simulink model "IEEE_9bus"  (R2023b)
settings: Solver=ode23tb  StartTime=0.0  StopTime=1  FixedStep=Ts  RelTol=1e-3
values from neighbouring files (symbols this model uses):
  N = 1    [IEEE_9bus_calc.m]
  Ts = 50e-6    (= 5e-05)    [IEEE_9bus_calc.m]
  Ws = 2*pi*f    (= 376.991118431)    [IEEE_9bus_calc.m]
undefined symbols (not defined in the file or in its folder): D1, Delta, DiscIntNeverNeededParam, SM, SYS
libraries: spsLoadFlowBusLib x9, spsabctodq0Lib x7, spsThreePhasePISectionLineLib x6, spsExcitationSystemLib x6, spsGenericPowerSystemStabilizerLib x6, spsHydraulicTurbineandGovernorLib x6, spsMultiBandPowerSystemStabilizerLib x6, spsThreePhaseVIMeasurementLib x5, spsThreePhaseSeriesRLCLoadLib x4, DQN_Lib x3, spsGroundLib x3, spsThreePhaseParallelRLCBranchLib x3
(part 1 of 3)
settings Model: Creator=z0034ktr  LastModifiedBy=rober
settings SolverCC: AlgebraicLoopSolver=TrustRegion  EnableFixedStepZeroCrossing=on
settings ModelReferenceCC: EnableRefExpFcnMdlSchedulingChecks=on

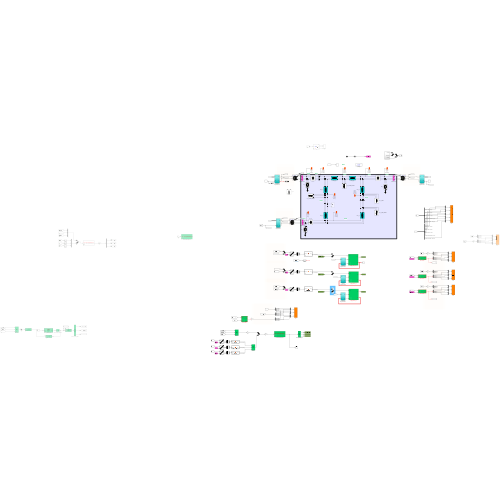
[thumbnail: Simulink's stored preview of the top-level diagram]
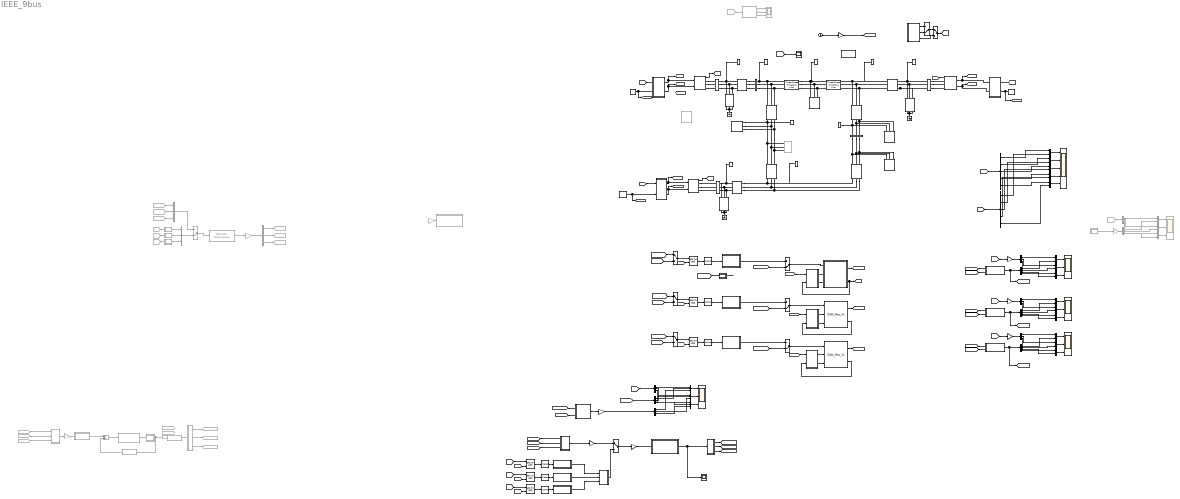
== system IEEE_9bus ==
  note: BUS7
  note: BUS7
  note: BUS2
  note: BUS8
  note: BUS9
  note: BUS3
  note: BUS6
  note: BUS4
  note: BUS5
  note: BUS1
  ABsel : Subsystem  Commented=on
  ABsel1 : Subsystem  Commented=on
  ABsel2 : Subsystem  Commented=on
  ABsel3 : Subsystem
  ABsel4 : Subsystem  Commented=on
  Add3 : Sum  Commented=on
  Bus Selector : BusSelector  OutputSignals="dq0 components.Stator voltage  vd (pu),dq0 components.Stator voltage  vq (pu),Mechanical.Rotor speed  wm  (pu),Mechanical.Rotor speed deviation  dw (pu),Output active power   Peo (pu)"
  Bus Selector1 : BusSelector  OutputSignals="Stator voltage  vd (pu),Stator voltage  vq (pu),Rotor speed  wm  (pu),Rotor speed deviation  dw (pu),Output active power   Peo (pu)"
  Clock : Clock
  Constant : Constant  Value=0.65694
  Constant1 : Constant  Value=0.825
  Constant2 : Constant  Value=0.425
  DQN_Mac1_V1 : Subsystem  mask{HRM=N, NomParam=[200E6  16500   60 ], reactVec=[ 1.305, 0.296, 0.252, 0.474, 0.243, 0.18 ], timeConstVec=[ 1.01, 0.053, 0.0513 ], Rs=2.8544e-3, Mech=[ 3.7 0  32], lfVec=[0.6569    0.3081    1.0000    1.5789   deg2rad(0)], Ts=Ts, SW=on, dbg=off, SMdbg=[]}
      mask prompts: HRM "Harmonic order:"; NomParam "Nominal power, line-to-line voltage, frequency [ Pn(VA)  Vn(Vrms)  fn(Hz) ]:"; reactVec "Reactances [ Xd  Xd'  Xd''  Xq  (Xq')  Xq''  Xl ] (pu):"; timeConstVec "[ Td'  Td''  (Tq')  Tq'' ] (s):"; Rs "Stator resistance Rs (pu):"; Mech "Inertia coefficient, friction factor, pole pairs [ H(s)  F(pu)  p()]:"; lfVec "Initial condition (P, Q, Vbus, Vf, angle) [1x6]:"; Ts "Integration timestep (s):"; SW "Method (dq - checked / abc - unchecked)"; dbg "Debug [external SM(RD) variable]"; SMdbg "Debug SM:"
      mask init:
      | SMRD = struct();
      | 
      |     SMRD.dwo = 0;
      | 
      |     SMRD.nState = numel(reactVec)-1;
      |     
      |     if(SMRD.nState>5)
      |         SMRD.RLinv   = zeros(6,6);
      |         SMRD.Linv    = zeros(6,6);
      |         SMRD.L       = zeros(6,6);
      |         SMRD.R       = zeros(6,6);
      |         W = zeros(6,6);
      |     else
      |         SMRD.RLinv   = zeros(5,5);
      |         SMRD.Linv    = zeros(5,5);
      |         SMRD.L       = zeros(5,5);
      |         SMRD.R       = zeros(5,5);
      |         W            = zeros(5,5);
      |     end
      | 
      |     SMRD.Rs      = Rs;
      | 
      |     SMRD.N       = 1;
      |     
      |     SMRD.H       = Mech(1);
      |     SMRD.F       = Mech(2);
      |     SMRD.p       = Mech(3);
      | 
      |     SMRD.Pn = NomParam(1);
      |     SMRD.Vn = NomParam(2);
      |     SMRD.fn = NomParam(3);
      |     
      |     
      |     Vb = SMRD.Vn*sqrt(2/3);
      |     Ib = sqrt(2/3)*SMRD.Pn/SMRD.Vn;
      |     
      |     
      |     Td_p    = timeConstVec(1);
      |     Td_pp   = timeConstVec(2);
      |     if(SMRD.nState>5)
      |         Tq_p    = timeConstVec(3);
      |         Tq_pp   = timeConstVec(4);
      |     else
      |         Tq_pp   = timeConstVec(3);
      |     end
      |     
      |     
      |     %Set the time constants in Lq(s)
      |     %See (eq. 7.2.14)
      |     
      |     wn=2*pi*SMRD.fn;
      |     SMRD.wn = wn;%Rated frequency in rad/sec
      |     %Implementation of the formulas in 
      |     
      |     % Xaq=1.165; %Mutual inductance
      |     % Ll=.188; %Stator leakage inductance
      |     
      |     %T5=0.0234;
      |     
      |     
      |     Xd      = reactVec(1);
      |     Xd_p    = reactVec(2);
      |     Xd_pp   = reactVec(3);
      |     Xq      = reactVec(4);
      | 
      | 
      |     if(SMRD.nState>5)
      |         Xq_p    = reactVec(5);
      |         Xq_pp   = reactVec(6);
      |         Xl      = reactVec(7);
      | 
      |         Tqo_p   = Tq_p * Xq/Xq_p;
      |         Tqo_pp  = Tq_pp * Xq_p/Xq_pp;
      |     else
      |         Xq_pp   = reactVec(5);
      |         Xl      = reactVec(6);
      |         Tqo_pp  = Tq_pp * Xq/Xq_pp;
      |     end
      | 
      | 
      |     Xad     = Xd-Xl; %Mutual inductance
      |     Xaq     = Xq-Xl; %Mutual inductance
      |     
      |     
      |     SMRD.Xd = Xd;
      |     SMRD.Xq = Xq;
      |     SMRD.Xl = Xl;
      |     SMRD.Xad = Xad;
      |     SMRD.Xaq = Xaq;
      |     
      |         
      |    
      |     LAM1 = sqrt(Xd^2*Xd_pp^2*(Td_p-Td_pp)^2+2*Td_p*Td_pp*Xd*Xd_p*Xd_pp*(Xd-2*Xd_p+Xd_pp)-2*Td_pp*Xd*Xd_p*Xd_pp*(Xd-Xd_p+Xd_pp)+Td_pp^2*Xd_pp^2*(Xd^2+Xd_pp^2));
      |     Tdo_p  = (Td_p*Xd*Xd_pp+LAM1+Td_pp*(Xd*Xd_p+Xd_p*Xd_pp-Xd*Xd_pp))/(2*Xd_p*Xd_pp);
      |     Tdo_pp = Xd*Td_p*Td_pp/(Xd_pp*Tdo_p);
      |     % 
      |     % Tqo_p   = Tq_p * Xq/Xq_p;
      |     % Tqo_pp  = Tq_pp * Xq_p/Xq_pp;
      | 
      | 
      |     % D-Axis
      |     a=SMRD.Xad*(Xd_p-SMRD.Xl)/(Xd-Xd_p);
      |     b=a*SMRD.Xad*(Xd_pp-SMRD.Xl)/(a*Xd+SMRD.Xl*SMRD.Xad-(a+SMRD.Xad)*Xd_pp);
      |     c=(b+a*SMRD.Xl*SMRD.Xad/(SMRD.Xl*SMRD.Xad+a*Xd))/Td_pp;
      |     
      |     T5 = b/c;
      | 
      |     if(1)
      |         a = Xad*(Xd_p-Xl)/(Xd-Xd_p);
      |         b = Xad*(Xd_pp-Xl)/(a*Xd+Xl*Xad-(a+Xad)*Xd_pp);
      |         c = (1/Td_pp)*(b-(a*Xl*Xad)/(Xl*Xad+a*Xd) );
      |         
      |         T11d = b/c;
      |     end
      | 
      |     
      |     if(1)
      |         %Set the time constants in Ld(s),sG(s)
      |         %See (eq. 7.2.4-7.2.5)
      |         T1 = Td_p; %T1=1.419; %Td'
      |         T2 = Td_pp; %T2=0.0669; %Td''
      |         T3 = Tdo_p; %T3=5.62; %Tdo'
      |         T4 = Tdo_pp; %T4=0.09; %Tdo''
      |         %T5 = T5; %T5=0.0234;
      |         Ld = Xd; %Ld= 1.104; %Synchronous inductance
      |         Ll = Xl; %Ll=0.198; %Stator leakage inductance
      |         Lad = Xad; %Lad=Ld-Ll; %Mutual inductance
      |         %Rated frequency in rad/sec
      |         %Implementation of the formulas in
      | 
      |         T5 = T11d;
      | 
      |         Ro=wn*Ld*(T3+T4-T1-T2);
      |         Ro=Lad*Lad/Ro;
      |         a=Ld*(T1+T2)-Ll*(T3+T4);a=a/Lad;
      |         b=Ld*T1*T2-Ll*T3*T4; b=b/Lad;
      |         c=(T3*T4-T1*T2)/(T3+T4-T1-T2);
      | 
      |         Lf1d=b-a*T5+T5*T5; %in p.u.
      |         Lf1d=Ro*Lf1d/(c-T5); %in p.u.
      |         Rfd=Ro*(Lf1d+Ro*(2*T5-a));
      |         Rfd=Rfd/(Lf1d+Ro*(T5+c-a));%in p.u.
      | 
      |         R1d=Ro*Rfd/(Rfd-Ro); %in p.u.
      |         %Inductances in p.u.
      |         L1d=R1d*T5; 
      |         L1d=L1d*wn;
      | 
      |         Lfd=Rfd*(a-T5-Lf1d/Ro); %in p.u.
      |         Lfd=Lfd*wn; 
      |         Lf1d=Lf1d*wn;
      | 
      |         SMRD.Lf1d = Lf1d;
      |         SMRD.Rfd = Rfd;
      |         SMRD.R1d = R1d;
      |         SMRD.L1d = L1d;
      |         SMRD.Lfd = Lfd;
      |     end
      | 
      | 
      |     %%%%%%%%%%%%%%%%%%%%%%%%% Q AXIS %%%%%%%%%%%%%%%%%%%%%%%%% Tqo′ Xq″ Xq SMRD.Xl 
      |     
      |     if(SMRD.nState>5)
      |         %conv(x,y)= polynomial multiplication
      |         N=conv([Tq_p 1],[Tq_pp 1]); 
      |         D=conv([Tqo_p 1],[Tqo_pp 1]);
      |         Nz=conv(N-D*SMRD.Xl/Xq,[Xaq/SMRD.wn 0]);
      |         Dz=D-N; Nz=Nz(1:3); Dz=Dz(1:2);
      |         Req=Nz(3)/Dz(2);
      |         Nz=Nz/Nz(3); Dz=Dz/Dz(2);
      |         %compute polynomial roots and sort them
      |         Tab=sort(abs(roots(Nz))); Tab=1./Tab;
      |         Tm=sort(abs(roots(Dz))); Tm=1/Tm(1);
      |         %Solve a system of two linear equa�tions
      |         x=[1 1;Tab(1) Tab(2)]\[1 ;Tm]/Req;
      |         %Results
      |         SMRD.R1q=1/x(1); 
      |         SMRD.L1q=SMRD.wn*SMRD.R1q*Tab(1); %in p.u.
      |         SMRD.R2q=1/x(2); 
      |         SMRD.L2q=SMRD.wn*SMRD.R2q*Tab(2); %in p.u.
      |     else
      |         N=conv([1],[Tq_pp 1]); 
      |         D=conv([1],[Tqo_pp 1]);
      |         Nz=conv(N-D*SMRD.Xl/Xq,[Xaq/SMRD.wn 0]);
      |         Dz=D-N; Nz=Nz(1:2); Dz=Dz(1:1);
      |         Req=Nz(2)/Dz(1);
      |         Nz=Nz/Nz(2); Dz=Dz/Dz(1);
      |         %compute polynomial roots and sort them
      |         Tab=sort(abs(roots(Nz))); Tab=1./Tab;
      |         Tm=1;
      |         %Solve a system of two linear equa�tions
      |         x=[1;Tab(1)]/Req;
      |         %Results
      |         SMRD.R1q=1/x(1); 
      |         SMRD.L1q=SMRD.wn*SMRD.R1q*Tab(1); %in p.u.
      |     end
      |     
      |     %%%%%%%%%%%%%%%%%%%%%%%%%%%%%%%%%%%%%%%%%%%%%%%%%%%%%%%%%%
      | 
      |     %%%%%%%%%%%%%%%%%%%%%%%%% R/L MAT %%%%%%%%%%%%%%%%%%%%%%%%%
      | 
      |     q_axis = 1;
      | 
      | 
      |     if(SMRD.nState>5) % D = 2,3,4 ; Q = 1,5,6
      | 
      |         if(q_axis)
      |             SMRD.L(2,2) = SMRD.Xd;  SMRD.L(2,3) = SMRD.Xad;                         SMRD.L(2,4) = SMRD.Xad; %D
      |             SMRD.L(3,2) = SMRD.Xad; SMRD.L(3,3) = SMRD.Xad + SMRD.Lf1d + SMRD.Lfd;  SMRD.L(3,4) = SMRD.Lf1d + SMRD.Xad; %D
      |             SMRD.L(4,2) = SMRD.Xad; SMRD.L(4,3) = SMRD.Xad + SMRD.Lf1d;             SMRD.L(4,4) = SMRD.Lf1d + SMRD.Xad + SMRD.L1d; %D
      | 
      |             SMRD.L(1,1) = SMRD.Xq;  SMRD.L(1,5) = SMRD.Xaq;                         SMRD.L(1,6) = SMRD.Xaq; %Q
      |             SMRD.L(5,1) = SMRD.Xaq; SMRD.L(5,5) = SMRD.Xaq + SMRD.L1q;              SMRD.L(5,6) = SMRD.Xaq; %Q
      |             SMRD.L(6,1) = SMRD.Xaq; SMRD.L(6,5) = SMRD.Xaq;                         SMRD.L(6,6) = SMRD.Xaq + SMRD.L2q; %Q
      | 
      | 
      |             SMRD.R(1,1) = Rs;
      |             SMRD.R(2,2) = Rs;
      |             SMRD.R(3,3) = SMRD.Rfd;
      |             SMRD.R(4,4) = SMRD.R1d;
      |             SMRD.R(5,5) = SMRD.R1q;
      |             SMRD.R(6,6) = SMRD.R2q;
      | 
      |         else
      |             SMRD.L(1,1) = SMRD.Xd;  SMRD.L(1,3) = SMRD.Xad;                         SMRD.L(1,5) = SMRD.Xad;
      |             SMRD.L(2,2) = SMRD.Xq;  SMRD.L(2,4) = SMRD.Xaq;                         SMRD.L(2,6) = SMRD.Xaq;
      |             SMRD.L(3,1) = SMRD.Xad; SMRD.L(3,3) = SMRD.Xad + SMRD.Lf1d + SMRD.Lfd;  SMRD.L(3,5) = SMRD.Lf1d + SMRD.Xad;
      |             SMRD.L(4,2) = SMRD.Xaq; SMRD.L(4,4) = SMRD.Xaq + SMRD.L1q;              SMRD.L(4,6) = SMRD.Xaq;
      |             SMRD.L(5,1) = SMRD.Xad; SMRD.L(5,3) = SMRD.Xad + SMRD.Lf1d;             SMRD.L(5,5) = SMRD.Lf1d + SMRD.Xad + SMRD.L1d;
      |             SMRD.L(6,2) = SMRD.Xaq; SMRD.L(6,4) = SMRD.Xaq;                         SMRD.L(6,6) = SMRD.Xaq  + SMRD.L2q;
      | 
      |             SMRD.R(1,1) = Rs;
      |             SMRD.R(2,2) = Rs;
      |             SMRD.R(3,3) = SMRD.Rfd;
      |             SMRD.R(4,4) = SMRD.R1q;
      |             SMRD.R(5,5) = SMRD.R1d;
      |             SMRD.R(6,6) = SMRD.R2q;
      |         end
      |     else
      | 
      |         if(q_axis)
      |             SMRD.L(2,2) = SMRD.Xd;  SMRD.L(2,3) = SMRD.Xad;                         SMRD.L(2,4) = SMRD.Xad;           %D
      |             SMRD.L(3,2) = SMRD.Xad; SMRD.L(3,3) = SMRD.Xad + SMRD.Lf1d + SMRD.Lfd;  SMRD.L(3,4) = SMRD.Lf1d + SMRD.Xad; %D
      |             SMRD.L(4,2) = SMRD.Xad; SMRD.L(4,3) = SMRD.Xad + SMRD.Lf1d;             SMRD.L(4,4) = SMRD.Lf1d + SMRD.Xad + SMRD.L1d;  %D
      |             
      |             SMRD.L(1,1) = SMRD.Xq;  SMRD.L(1,5) = SMRD.Xaq;              %Q
      |             SMRD.L(5,1) = SMRD.Xaq; SMRD.L(5,5) = SMRD.Xaq + SMRD.L1q;   %Q
      | 
      |             SMRD.R(1,1) = Rs;
      |             SMRD.R(2,2) = Rs;
      |             SMRD.R(3,3) = SMRD.Rfd;
      |             SMRD.R(4,4) = SMRD.R1d;
      |             SMRD.R(5,5) = SMRD.R1q;
      | 
      |         else
      |             SMRD.L(1,1) = SMRD.Xd; SMRD.L(1,3) = SMRD.Xad; SMRD.L(1,5) = SMRD.Xad;
      |             SMRD.L(2,2) = SMRD.Xq; SMRD.L(2,4) = SMRD.Xaq;
      |             SMRD.L(3,1) = SMRD.Xad; SMRD.L(3,3) = SMRD.Xad + SMRD.Lf1d + SMRD.L1d; SMRD.L(3,5) = SMRD.Lf1d + SMRD.Xad;
      |             SMRD.L(4,2) = SMRD.Xaq; SMRD.L(4,4) = SMRD.Xaq + SMRD.L1q; 
      |             SMRD.L(5,1) = SMRD.Xad; SMRD.L(5,3) = SMRD.Xad + SMRD.Lf1d; SMRD.L(5,5) = SMRD.Lf1d + SMRD.Xad + SMRD.Lfd;
      | 
      |             SMRD.R(1,1) = Rs;
      |             SMRD.R(2,2) = Rs;
      |             SMRD.R(3,3) = SMRD.Rfd;
      |             SMRD.R(4,4) = SMRD.R1q;
      |             SMRD.R(5,5) = SMRD.R1d;
      | 
      |         end
      |     end
      | 
      | 
      |    if(q_axis)
      |         W(2,1) = -1;
      |         W(1,2) = +1;
      |    else
      |         W(2,1) = +1;
      |         W(1,2) = -1;
      |    end
      |     
      |     %%%%%%%%%%%%%%%%%%%%%%%%%%%%% LF  %%%%%%%%%%%%%%%%%%%%%%%%%
      |     
      |     Pt = lfVec(1);
      |     Qt = lfVec(2);
      |     Vt = lfVec(3);
      |     Et = lfVec(4);
      |     At = lfVec(5);
      |     % if(numel(lfVec)>5) fac = lfVec(6); end
      |     
      |     phi = At;
      |     SMRD.phi = phi;
      | 
      |     SMRD.Vt = Vt*exp(1i*(phi));
      |     SMRD.It = (Pt-1i*Qt)/(Vt*exp(-1i*(phi)));
      |        
      |     %fi = sign(Qt)*acos(Pt/(Vt*It)); rad2deg(fi);
      |     fi = angle(SMRD.Vt)-angle(SMRD.It);
      |     SMRD.fi = fi;
      |     
      |     % del = (atan((Xq*It*cos(fi)-Rs*It*sin(fi))/(Vt+Rs*It*cos(fi)+Xq*It*sin(fi))));
      |     del = angle(SMRD.Vt+(SMRD.Rs+1i*SMRD.Xq)*SMRD.It)-(SMRD.phi);
      | 
      |     SMRD.del = del;
      | 
      |     if(0) %Calculate Vfnp without p.u.
      |         SMRD.Vfnp = ((SMRD.Rfd*Vb/(Xad*wn))^2);
      |     else
      |         SMRD.Vfnp = SMRD.Rfd/SMRD.Xad;
      |     end
      |     
      |     v_dq = Vt*exp(1i*(pi/2-del)); %correct
      |     ed = real(v_dq);
      |     eq = imag(v_dq);
      |     efd = Et*SMRD.Vfnp;
      |     
      |    if(q_axis)
      |         v_vec = [eq; ed; efd; zeros(SMRD.nState-3,1)];
      |         i_vec = (v_vec'/(SMRD.R-SMRD.L*W))';
      |    else
      |         v_vec = [ed; eq; efd; zeros(SMRD.nState-3,1)];
      |         i_vec = (v_vec'/(SMRD.R-SMRD.L*W))';
      |    end
      | 
      |     %%%%%%%%%%%%%%%%%%%%%%%%%%%%%%%%%%%%%%%%%%%%%%%%%%%%%%%%%%
      |     
      |     SMRD.idq0 = i_vec;
      |     SMRD.phidq0 = SMRD.L*i_vec;
      |     
      |     SMRD.dwo = 0;
      | 
      |     SMRD.Linv = eye(SMRD.nState)/SMRD.L;
      |     
      |     if(1)
      |         SMRD.Linv2 = SMRD.Linv;
      |         SMRD.Linv2(3,4) = 0; SMRD.Linv2(4,3) = 0;
      |     end
      | 
      | 
      |     SMRD.RLinv = SMRD.R*SMRD.Linv;
      | 
      | 
      |     SMRD.Pb = 1;
      |     SMRD.Ib = Ib;
      |     SMRD.Vb = Vb;
      | 
      |     SMRD.IqdSign = [-1    -1     ones(1,SMRD.nState-2)];
      | 
      | 
      | 
      |     SMRD.web = SMRD.wn;
      |     SMRD.v_dq = v_dq;
      | 
      |     tho = del+phi-pi/2;
      |     SMRD.tho = tho;
      | 
      |     if(dbg && ~isempty(SMdbg))
      |         SMRD = SMdbg;
      |         SMRD.phidq0 = SMdbg.phiqd0;
      |         SMRD.N = HRM;
      |     end
      |         
      |     SMRD.Ts = Ts;
      settings: LibrarySourceBlock=|
      | spsSynchronousMachineModel/Continuous/Synchronous Machine
      | Continuous Model
      mask Callback dbg:
      | EMT = get_param(gcb,'dbg');
      | 
      |     if(strcmp(EMT,'on'))
      |        set_param(gcb,'MaskVisibilities',{'on','on','on','on','on','on','on','on','on','on','on'});
      |     else
      |        set_param(gcb,'MaskVisibilities',{'on','on','on','on','on','on','on','on','on','on','off'});
      |     end
  DQN_Mac2_V1 : DQN_Machines/DQN_Mac_V1  HRM=N  NomParam="[200E6  18000   60 ]"  reactVec=[ 1.305, 0.296, 0.252, 0.474, 0.243, 0.18 ]  timeConstVec=[ 1.01, 0.053, 0.0513 ]  Rs=2.8544e-3  Mech="[ 3.7 0  32]"  lfVec="[0.8250    0.2219    1.0000    1.5762   deg2rad(6.37)]"  Ts=Ts  SW=on  dbg=off  SMdbg=[]
      settings: LibrarySourceBlock=|
      | spsSynchronousMachineModel/Continuous/Synchronous Machine
      | Continuous Model
  DQN_Mac3_V1 : DQN_Machines/DQN_Mac_V1  HRM=N  NomParam="[200E6  13800   60 ]"  reactVec=[ 1.305, 0.296, 0.252, 0.474, 0.243, 0.18 ]  timeConstVec=[ 1.01, 0.053, 0.0513 ]  Rs=2.8544e-3  Mech="[ 3.7 0  32]"  lfVec="[0.4250    0.1355    1.0000    1.2604  deg2rad(-0.3643)]"  Ts=Ts  SW=on  dbg=off  SMdbg=[]
      settings: LibrarySourceBlock=|
      | spsSynchronousMachineModel/Continuous/Synchronous Machine
      | Continuous Model
  DQn->ABC1 : MATLAB Function  TreatAsAtomicUnit=on  mask{N=N}
      mask prompts: N "Harmonic order:"
  DQn->ABC2 : MATLAB Function  TreatAsAtomicUnit=on  mask{N=N}
      mask prompts: N "Harmonic order:"
  DQn->ABC3 : MATLAB Function  TreatAsAtomicUnit=on  mask{N=N}
      mask prompts: N "Harmonic order:"
  DQn->ABC4 : MATLAB Function  TreatAsAtomicUnit=on  SystemSampleTime=Ts  mask{N=N}
      mask prompts: N "Harmonic order:"
  Demux : Demux  Commented=on  Outputs=3
  Demux1 : Demux  Commented=on  Outputs=3
  Demux{5..11,46..47} (9 alike) : Demux  Outputs=3
  Demux2 : Demux  Commented=on  Outputs=3
  Demux_DQNc_Mat : Subsystem  mask{nrOut=3}
      mask prompts: nrOut "Number of outputs [{C}]"
      mask init:
      | if(isempty(nrOut))
      |     Simulink.SubSystem.deleteContents(gcb);
      | else
      | 
      |     IndexOptionArray = cell(2,1);
      |     IndexOptionArray(1) = {'Select all'           };
      |     IndexOptionArray(2) = {'Index vector (dialog)'};
      | 
      |     PortHandles = get_param(gcb,'PortHandles');
      | 
      |     lenOut = length(PortHandles.Outport);
      | 
      |     if(nrOut ~= lenOut) % Important to avoid reinitialization of the block!
      | 
      |         Simulink.SubSystem.deleteContents(gcb);
      | 
      |         add_block('built-in/Inport',[gcb,strcat('/In',num2str(1))]);
      |         set_param([gcb,strcat('/In',num2str(1))],'position' , [50,65+1*50,90,85+1*50]);
      | 
      |         for i = 1 : nrOut
      |             add_block('simulink/Signal Routing/Selector',[gcb,strcat('/Sel',num2str(i))],...
      |                 'IndexOptionArray',IndexOptionArray,...
      |                 'NumberOfDimensions','2',...
      |                 'IndexOptions','Index vector (dialog),Select all',...
      |                 'Indices',strcat(num2str((i-1)*3+1),':',num2str((i-1)*3+3),', 1') ...
      |                 );
      |             set_param([gcb,strcat('/Sel',num2str(i))],'position' , [450,65+i*50,490,85+i*50])
      | 
      | 
      |             add_block('built-in/Outport',[gcb,strcat('/Out',num2str(i))]);
      |             set_param([gcb,strcat('/Out',num2str(i))],'position' , [750,65+i*50,790,85+i*50]);
      | 
      |             add_line(gcb,strcat('In',num2str(1),'/1'),  strcat('Sel',num2str(i),'/1'),'autorouting','on');
      |             add_line(gcb,strcat('Sel',num2str(i),'/1'), strcat('Out',num2str(i),'/1'),'autorouting','on');
      |         end
      | 
      |     end
      | 
      | end
      mask Display: disp(['{\color{red}\bf\fontsize{12}} [\{X_C\}]',newline,' DE-',newline,' MUX'], 'texmode','on');
  Demux_DQNc_Mat2 : Subsystem  Commented=on  mask{nrOut=3}
      mask prompts: nrOut "Number of outputs [{C}]"
      mask init: same as IEEE_9bus/Demux_DQNc_Mat
      mask Display: disp(['{\color{red}\bf\fontsize{12}} [\{X_C\}]',newline,' DE-',newline,' MUX'], 'texmode','on');
  Discrete State-Space1 : DQN_Lib/Discrete State-Space  Commented=on  A=SYS.A  B=SYS.B  C=SYS.C  D=SYS.D  InitVec=SYS.x0  dt=Ts
      settings: LibrarySourceBlock=|
      | spsSynchronousMachineModel/Discrete robust/State Space Model/Discretize
      | BE or Tustin
  Discrete State-Space2 : Subsystem  mask{A=SYS.A, B=SYS.B, C=SYS.C, D=SYS.D, InitVec=SYS.x0, dt=Ts, N=N, Ws=Ws}
      mask prompts: InitVec "Initial condition:"; dt "Time step (s):"; N "Order number:"; Ws "Angular frequency (rad/s);"
      mask init:
      | %Discretization of Continuous-Time Systems in the State Space with Numerical Integration Methods
      | 
      | method = 0;
      | 
      | if(method)
      | 
      |     I = eye(size(A,1));
      |     INVR = I/(I-A*dt/2);
      |     Ad1 = INVR*(I+A*dt/2);
      |     Bd1 = INVR*B*dt/2;
      |     Cd1 = C*Ad1;
      |     Dd1 = C*INVR*B*dt/2+D;
      |     Dd12 = C*INVR*B*dt/2;
      | 
      | else
      |     I = eye(size(A,1));
      |     INVR = I/(I-A*dt/2);
      |     Ad1 = INVR*(I+A*dt/2);
      |     Bd1 = INVR*B;
      |     Cd1 = C*INVR*dt;
      |     Dd1 = Cd1*B/2;
      | end
      | 
      | %Calculating the PNZ matrices
      | 
      |     a = -0.5+0.866i;
      |     a2 = -0.5-0.866i;
      |     Sas = [1,a,a2;1,a2,a;1,1,1]/3;
      | 
      |     arows = size(Ad1,1)/3; %signal size
      |     acols = size(Ad1,2)/3; %signal size
      | 
      |     brows = size(Bd1,1)/3; %signal size
      |     bcols = size(Bd1,2)/3; %signal size
      | 
      |     crows = size(Cd1,1)/3; %signal size
      |     ccols = size(Cd1,2)/3; %signal size
      | 
      |     d1rows = size(Dd1,1)/3; %signal size
      |     d1cols = size(Dd1,2)/3; %signal size
      | 
      |     if(method)
      |         d2rows = size(Dd12,1)/3; %signal size
      |         d2cols = size(Dd12,2)/3; %signal size
      |     end
      | 
      | 
      |     %%%%%%%%%%%%%%%%%%%%%%% Check for inconsistencies  %%%%%%%%%%%%%%%%%%%%%%%
      | 
      |     szMatA = size(A,1);
      |     iL = eye(szMatA);
      |     szMatiL = size(iL,1);
      | 
      |     if(szMatiL ~= szMatA || size(A,1) ~= size(A,2) || size(iL,1) ~= size(iL,2))
      |         error('[Int_DQN_Mat/swFeedback] check matrix A size!');
      |     end
      | 
      |     if(arows ~= brows || acols ~= ccols || crows ~= d1rows || bcols ~= d1cols)
      |         error('[Int_DQN_Mat/Initialize] the sizes of the state-space matrices!');
      |     end
      | 
      |     %%%%%%%%%%%%%%%%%%%%%%%%%%%%%%%%%%%%%%%%%%%%%%%%%%%%%%%%%%%%%%%
      | 
      | 
      |     %%%%%%%%%%%%%%%%%%%%%%% A --> Bpnz %%%%%%%%%%%%%%%%%%%%%%%
      |     Adc = complex(zeros(3*arows,3*acols));
      | 
      |     for i = 1 : arows
      |         for j = 1 : acols
      |             Adc((1:3) + (i-1)*3,(1:3) + (j-1)*3) = Sas*Ad1((1:3) + (i-1)*3,(1:3) + (j-1)*3)/Sas;
      |             %Adc((1:3) + (i-1)*3,(1:3) + (j-1)*3) = diag(diag(real(Adc((1:3) + (i-1)*3,(1:3) + (j-1)*3))));
      |         end
      |     end
      |     %%%%%%%%%%%%%%%%%%%%%%%%%%%%%%%%%%%%%%%%%%%%%%%%%%%%%%%%%%%%%%%
      | 
      |     %%%%%%%%%%%%%%%%%%%%%%% B --> Bpnz %%%%%%%%%%%%%%%%%%%%%%%
      | 
      |     Bdc = complex(zeros(3*brows,3*bcols));
      | 
      |     for i = 1 : brows
      |         for j = 1 : bcols
      |             Bdc((1:3) + (i-1)*3,(1:3) + (j-1)*3) = Sas*Bd1((1:3) + (i-1)*3,(1:3) + (j-1)*3)/Sas;
      |             %Bdc((1:3) + (i-1)*3,(1:3) + (j-1)*3) = diag(diag(real(Bdc((1:3) + (i-1)*3,(1:3) + (j-1)*3))));
      |         end
      |     end
      |     %%%%%%%%%%%%%%%%%%%%%%%%%%%%%%%%%%%%%%%%%%%%%%%%%%%%%%%%%%%%%%%
      | 
      |     %%%%%%%%%%%%%%%%%%%%%%% C --> Cpnz %%%%%%%%%%%%%%%%%%%%%%%
      | 
      |     Cdc = complex(zeros(3*crows,3*ccols));
      | 
      |     for i = 1 : crows
      |         for j = 1 : ccols
      |             Cdc((1:3) + (i-1)*3,(1:3) + (j-1)*3) = Sas*Cd1((1:3) + (i-1)*3,(1:3) + (j-1)*3)/Sas;
      |             %Cdc((1:3) + (i-1)*3,(1:3) + (j-1)*3) = diag(diag(real(Cdc((1:3) + (i-1)*3,(1:3) + (j-1)*3))));
      |         end
      |     end
      |     %%%%%%%%%%%%%%%%%%%%%%%%%%%%%%%%%%%%%%%%%%%%%%%%%%%%%%%%%%%%%%%
      | 
      |     
      |     %%%%%%%%%%%%%%%%%%%%%%% D1 --> Cpnz %%%%%%%%%%%%%%%%%%%%%%%
      | 
      |     Ddc = complex(zeros(3*d1rows,3*d1cols));
      | 
      |     for i = 1 : d1rows
      |         for j = 1 : d1cols
      |             Ddc((1:3) + (i-1)*3,(1:3) + (j-1)*3) = Sas*Dd1((1:3) + (i-1)*3,(1:3) + (j-1)*3)/Sas;
      |             %Ddc1((1:3) + (i-1)*3,(1:3) + (j-1)*3) = diag(diag(real(Ddc1((1:3) + (i-1)*3,(1:3) + (j-1)*3))));
      |         end
      |     end
      |     %%%%%%%%%%%%%%%%%%%%%%%%%%%%%%%%%%%%%%%%%%%%%%%%%%%%%%%%%%%%%%%
      | 
      | if(method)
      |     %%%%%%%%%%%%%%%%%%%%%%% D2 --> Cpnz %%%%%%%%%%%%%%%%%%%%%%%
      | 
      |     Ddc2 = complex(zeros(3*d2rows,3*d2cols));
      | 
      |     for i = 1 : d2rows
      |         for j = 1 : d2cols
      |             Ddc2((1:3) + (i-1)*3,(1:3) + (j-1)*3) = Sas*Dd12((1:3) + (i-1)*3,(1:3) + (j-1)*3)/Sas;
      |             %Ddc2((1:3) + (i-1)*3,(1:3) + (j-1)*3) = diag(diag(real(Ddc2((1:3) + (i-1)*3,(1:3) + (j-1)*3))));
      |         end
      |     end
      |     %%%%%%%%%%%%%%%%%%%%%%%%%%%%%%%%%%%%%%%%%%%%%%%%%%%%%%%%%%%%%%%
      | 
      | end
      | 
      |     % Adc(abs(Adc)<10*eps) = 0;
      |     % Bdc(abs(Bdc)<10*eps) = 0;
      |     % Cdc(abs(Cdc)<10*eps) = 0;
      |     % Ddc(abs(Ddc)<10*eps) = 0;
      | 
      |     InitVec_c = complex(zeros(brows*3,N+1));
      | 
      | 
      |     if(~isempty(InitVec))
      |         if(mod(numel(InitVec),3)~=0) error('[SS_DQNc_Mat] InitVec with wrong size --> needs to be a multiple of 3!'); end
      | 
      |         for k = 1 : numel(InitVec)/3
      |             InitVec_c((k-1)*3+1:(k-1)*3+3,1) = Sas*InitVec((k-1)*3+1:(k-1)*3+3)*exp(+1i*Ws*dt);
      |         end
      |     end
      settings: LibrarySourceBlock=|
      | spsSynchronousMachineModel/Discrete robust/State Space Model/Discretize
      | BE or Tustin
      mask Display: disp(['{\color{red}\bf\fontsize{12}x(t) = Ad*x(t-dt)+Bd*u(t)}',newline,'{\color{gray}\bf\fontsize{12}y(t) = Cd*x(t-dt)+Dd*u(t)}'], 'texmode','on');
  Discrete State-Space3 : Subsystem  Commented=on  mask{A=SYS.A, B=SYS.B, C=SYS.C, D=SYS.D, InitVec=SYS.x0, dt=Ts, N=N}
      mask prompts: InitVec "Initial condition:"; dt "Time step (s):"; N "Order number:"
      mask init:
      | %Discretization of Continuous-Time Systems in the State Space with Numerical Integration Methods
      | 
      | I = eye(size(A,1));
      | INVR = I/(I-A*dt/2);
      | Ad1 = INVR*(I+A*dt/2);
      | Bd1 = INVR*B*dt/2;
      | Cd1 = C*Ad1;
      | Dd11 = C*INVR*B*dt/2+D;
      | Dd12 = C*INVR*B*dt/2;
      | 
      | %Calculating the PNZ matrices
      | 
      |     a = -0.5+0.866i;
      |     a2 = -0.5-0.866i;
      |     Sas = [1,a,a2;1,a2,a;1,1,1]/3;
      | 
      |     arows = size(Ad1,1)/3; %signal size
      |     acols = size(Ad1,2)/3; %signal size
      | 
      |     brows = size(Bd1,1)/3; %signal size
      |     bcols = size(Bd1,2)/3; %signal size
      | 
      |     crows = size(Cd1,1)/3; %signal size
      |     ccols = size(Cd1,2)/3; %signal size
      | 
      |     d1rows = size(Dd11,1)/3; %signal size
      |     d1cols = size(Dd11,2)/3; %signal size
      | 
      |     d2rows = size(Dd12,1)/3; %signal size
      |     d2cols = size(Dd12,2)/3; %signal size
      | 
      | 
      |     %%%%%%%%%%%%%%%%%%%%%%% Check for inconsistencies  %%%%%%%%%%%%%%%%%%%%%%%
      | 
      |     szMatA = size(A,1);
      |     iL = eye(szMatA);
      |     szMatiL = size(iL,1);
      | 
      |     if(szMatiL ~= szMatA || size(A,1) ~= size(A,2) || size(iL,1) ~= size(iL,2))
      |         error('[Int_DQN_Mat/swFeedback] check matrix A size!');
      |     end
      | 
      |     if(arows ~= brows || acols ~= ccols || crows ~= d1rows || bcols ~= d1cols)
      |         error('[Int_DQN_Mat/Initialize] the sizes of the state-space matrices!');
      |     end
      | 
      |     %%%%%%%%%%%%%%%%%%%%%%%%%%%%%%%%%%%%%%%%%%%%%%%%%%%%%%%%%%%%%%%
      | 
      | 
      |     %%%%%%%%%%%%%%%%%%%%%%% A --> Bpnz %%%%%%%%%%%%%%%%%%%%%%%
      |     Adc = complex(zeros(3*arows,3*acols));
      | 
      |     for i = 1 : arows
      |         for j = 1 : acols
      |             Adc((1:3) + (i-1)*3,(1:3) + (j-1)*3) = Sas*Ad1((1:3) + (i-1)*3,(1:3) + (j-1)*3)/Sas;
      |             %Adc((1:3) + (i-1)*3,(1:3) + (j-1)*3) = diag(diag(real(Adc((1:3) + (i-1)*3,(1:3) + (j-1)*3))));
      |         end
      |     end
      |     %%%%%%%%%%%%%%%%%%%%%%%%%%%%%%%%%%%%%%%%%%%%%%%%%%%%%%%%%%%%%%%
      | 
      |     %%%%%%%%%%%%%%%%%%%%%%% B --> Bpnz %%%%%%%%%%%%%%%%%%%%%%%
      | 
      |     Bdc = complex(zeros(3*brows,3*bcols));
      | 
      |     for i = 1 : brows
      |         for j = 1 : bcols
      |             Bdc((1:3) + (i-1)*3,(1:3) + (j-1)*3) = Sas*Bd1((1:3) + (i-1)*3,(1:3) + (j-1)*3)/Sas;
      |             %Bdc((1:3) + (i-1)*3,(1:3) + (j-1)*3) = diag(diag(real(Bdc((1:3) + (i-1)*3,(1:3) + (j-1)*3))));
      |         end
      |     end
      |     %%%%%%%%%%%%%%%%%%%%%%%%%%%%%%%%%%%%%%%%%%%%%%%%%%%%%%%%%%%%%%%
      | 
      |     %%%%%%%%%%%%%%%%%%%%%%% C --> Cpnz %%%%%%%%%%%%%%%%%%%%%%%
      | 
      |     Cdc = complex(zeros(3*crows,3*ccols));
      | 
      |     for i = 1 : crows
      |         for j = 1 : ccols
      |             Cdc((1:3) + (i-1)*3,(1:3) + (j-1)*3) = Sas*Cd1((1:3) + (i-1)*3,(1:3) + (j-1)*3)/Sas;
      |             %Cdc((1:3) + (i-1)*3,(1:3) + (j-1)*3) = diag(diag(real(Cdc((1:3) + (i-1)*3,(1:3) + (j-1)*3))));
      |         end
      |     end
      |     %%%%%%%%%%%%%%%%%%%%%%%%%%%%%%%%%%%%%%%%%%%%%%%%%%%%%%%%%%%%%%%
      | 
      |     %%%%%%%%%%%%%%%%%%%%%%% D1 --> Cpnz %%%%%%%%%%%%%%%%%%%%%%%
      | 
      |     Ddc1 = complex(zeros(3*d1rows,3*d1cols));
      | 
      |     for i = 1 : d1rows
      |         for j = 1 : d1cols
      |             Ddc1((1:3) + (i-1)*3,(1:3) + (j-1)*3) = Sas*Dd11((1:3) + (i-1)*3,(1:3) + (j-1)*3)/Sas;
      |             %Ddc1((1:3) + (i-1)*3,(1:3) + (j-1)*3) = diag(diag(real(Ddc1((1:3) + (i-1)*3,(1:3) + (j-1)*3))));
      |         end
      |     end
      |     %%%%%%%%%%%%%%%%%%%%%%%%%%%%%%%%%%%%%%%%%%%%%%%%%%%%%%%%%%%%%%%
      | 
      |     %%%%%%%%%%%%%%%%%%%%%%% D2 --> Cpnz %%%%%%%%%%%%%%%%%%%%%%%
      | 
      |     Ddc2 = complex(zeros(3*d2rows,3*d2cols));
      | 
      |     for i = 1 : d2rows
      |         for j = 1 : d2cols
      |             Ddc2((1:3) + (i-1)*3,(1:3) + (j-1)*3) = Sas*Dd12((1:3) + (i-1)*3,(1:3) + (j-1)*3)/Sas;
      |             %Ddc2((1:3) + (i-1)*3,(1:3) + (j-1)*3) = diag(diag(real(Ddc2((1:3) + (i-1)*3,(1:3) + (j-1)*3))));
      |         end
      |     end
      |     %%%%%%%%%%%%%%%%%%%%%%%%%%%%%%%%%%%%%%%%%%%%%%%%%%%%%%%%%%%%%%%
      | 
      |     % Adc(abs(Adc)<10*eps) = 0;
      |     % Bdc(abs(Bdc)<10*eps) = 0;
      |     % Cdc(abs(Cdc)<10*eps) = 0;
      |     % Ddc(abs(Ddc)<10*eps) = 0;
      | 
      |     InitVec_c = complex(zeros(brows*3,N+1));
      | 
      | 
      |     if(~isempty(InitVec))
      |         if(mod(numel(InitVec),3)~=0) error('[SS_DQNc_Mat] InitVec with wrong size --> needs to be a multiple of 3!'); end
      | 
      |         for k = 1 : numel(InitVec)/3
      |             InitVec_c((k-1)*3+1:(k-1)*3+3,1) = Sas*InitVec((k-1)*3+1:(k-1)*3+3);
      |         end
      |     end
      settings: LibrarySourceBlock=|
      | spsSynchronousMachineModel/Discrete robust/State Space Model/Discretize
      | BE or Tustin
      mask Display: disp(['{\color{red}\bf\fontsize{12}x(t) = Ad*x(t-dt)+Bd*u(t)}',newline,'{\color{gray}\bf\fontsize{12}y(t) = Cd*x(t-dt)+Dd*u(t)}'], 'texmode','on');
  From : From  Commented=on  GotoTag=Vabc_B9  TagVisibility=global
  From23 : From  Commented=on  GotoTag=Im1_C
  From32 : From  Commented=on  GotoTag=Im2_C
  From33 : From  Commented=on  GotoTag=Im3_C
  From48 : From  Commented=on  GotoTag=Im1_abc
  From5 : From  Commented=on  GotoTag=IBUS1  TagVisibility=global
  From50 : From  Commented=on  GotoTag=Im2_abc
  From53 : From  Commented=on  GotoTag=Im3_abc
  From55 : From  Commented=on  GotoTag=Im1_C
  From56 : From  Commented=on  GotoTag=IBUS1  TagVisibility=global
  From57 : From  Commented=on  GotoTag=Im2_C
  From58 : From  Commented=on  GotoTag=Im3_C
  From6 : From  Commented=on  GotoTag=IBUS2  TagVisibility=global
  From7 : From  Commented=on  GotoTag=IBUS3  TagVisibility=global
  Gain : Gain
  Gain{1..3,9} (4 alike) : Gain  Commented=on  Gain=-1
  Gain12 : Gain  Gain=Ws
  Gain{4..8} (5 alike) : Gain  Gain=-1
  Gain_DQNc_Mat1 : DQN_Lib/Gain_DQNc_Mat  Commented=on  Rabc=SYS.C  HRM=N  chkInv=off
  Gain_DQNc_Mat4 : MATLAB Function  Commented=on  TreatAsAtomicUnit=on  SystemSampleTime=Ts  mask{Rabc=SYS.B, HRM=N, chkInv=off}
      mask prompts: Rabc "Line matrix [3x3]:"; HRM "Harmonic order:"; chkInv "Invert"
  Gain_DQNc_Mat5 : DQN_Lib/Gain_DQNc_Mat  Commented=on  Rabc=SYS.A  HRM=N  chkInv=off
  Goto10 : Goto  Commented=on  GotoTag=VBUS1_C
  Goto13 : Goto  Commented=on  GotoTag=VBUS2_C
  Goto14 : Goto  Commented=on  GotoTag=VBUS3_C
  Goto4 : Goto  Commented=on  GotoTag=VBUS1_SS
  Goto5 : Goto  Commented=on  GotoTag=VBUS2_SS
  Goto6 : Goto  Commented=on  GotoTag=VBUS3_SS
  Ground : spsGroundLib/Ground  LConnTagsString=a
  Ground1 : spsGroundLib/Ground  LConnTagsString=a
  Ground2 : spsGroundLib/Ground  LConnTagsString=a
  Int_DQNc_Mat3 : MATLAB Function  Commented=on  TreatAsAtomicUnit=on  mask{N=N, dt=Ts, w=Ws, InitInt=SYS.x0, swFeed=off, R=-SYS.A, iL=eye(size(SYS.A,1))}
      mask prompts: N "Order number:"; dt "Time step (s):"; w "Angular frequency (1/rad):"; InitInt "Initial conditions DC [3x1]:"; swFeed "Enable feedback"; R "Feedback parameter (Kr {abc}):"; iL "Feedback parameter (Ki {abc}):"
  LD_1 : spsThreePhaseParallelRLCBranchLib/Three-Phase Parallel RLC Branch  LConnTagsString=A|B|C  RConnTagsString=A|B|C  BranchType=RC  Resistance=(16.5e3)^2/2e6  Inductance=1e-3  Capacitance=1/(Ws*(16.5e3)^2/2e6)  Measurements=None
  LD_2 : spsThreePhaseParallelRLCBranchLib/Three-Phase Parallel RLC Branch  LConnTagsString=A|B|C  RConnTagsString=A|B|C  BranchType=RC  Resistance=(18e3)^2/2e6  Inductance=1e-3  Capacitance=1/(Ws*(18e3)^2/2e6)  Measurements=None
  LD_22 : spsThreePhaseParallelRLCLoadLib/Three-Phase Parallel RLC Load  Commented=on  LConnTagsString=A|B|C  Configuration=Y (grounded)  NominalVoltage=18e3  Vabc=[1e3 1e3 1e3]  Vabcp=[1e3 1e3 1e3]  NominalFrequency=60  UnbalancedPower=off  ActivePower=10000  InductivePower=0  CapacitivePower=0  Pabc=[10e3 9e3 11e3]  QLabc=[100 90 110]  QCabc=[100 90 110]  Pabcp=[10e3 9e3 11e3]  QLabcp=[100 90 110]  QCabcp=[100 90 110]  Measurements=None  LoadType=constant Z
  LD_3 : spsThreePhaseParallelRLCBranchLib/Three-Phase Parallel RLC Branch  LConnTagsString=A|B|C  RConnTagsString=A|B|C  BranchType=RC  Resistance=(16.5e3)^2/2e6  Inductance=1e-3  Capacitance=1/(Ws*(16.5e3)^2/2e6)  Measurements=None
  LD_5_125MW_50MVAr : spsThreePhaseSeriesRLCLoadLib/Three-Phase Series RLC Load  LConnTagsString=A|B|C  Configuration=Y (grounded)  NominalVoltage=(230000)*0.903808  Vabc=[1e3 1e3 1e3]  Vabcp=[1e3 1e3 1e3]  NominalFrequency=60  UnbalancedPower=off  ActivePower=125000000  InductivePower=50000000  CapacitivePower=0  Pabc=[10e3 9e3 11e3]  QLabc=[100 90 110]  QCabc=[100 90 110]  Pabcp=[10e3 9e3 11e3]  QLabcp=[100 90 110]  QCabcp=[100 90 110]  Measurements=None  LoadType=constant PQ
  LD_6_50MW : spsThreePhaseSeriesRLCLoadLib/Three-Phase Series RLC Load  LConnTagsString=A|B|C  Configuration=Y (grounded)  NominalVoltage=(230000)*0.916316  Vabc=[1e3 1e3 1e3]  Vabcp=[1e3 1e3 1e3]  NominalFrequency=60  UnbalancedPower=off  ActivePower=50000000  InductivePower=0  CapacitivePower=0  Pabc=[10e3 9e3 11e3]  QLabc=[100 90 110]  QCabc=[100 90 110]  Pabcp=[10e3 9e3 11e3]  QLabcp=[100 90 110]  QCabcp=[100 90 110]  Measurements=None  LoadType=constant PQ
  LD_6_90MW_30MVAr : spsThreePhaseSeriesRLCLoadLib/Three-Phase Series RLC Load  LConnTagsString=A|B|C  Configuration=Y (grounded)  NominalVoltage=(230000)*0.916316  Vabc=[1e3 1e3 1e3]  Vabcp=[1e3 1e3 1e3]  NominalFrequency=60  UnbalancedPower=off  ActivePower=90000000  InductivePower=30000000  CapacitivePower=0  Pabc=[10e3 9e3 11e3]  QLabc=[100 90 110]  QCabc=[100 90 110]  Pabcp=[10e3 9e3 11e3]  QLabcp=[100 90 110]  QCabcp=[100 90 110]  Measurements=None  LoadType=constant PQ
  LD_8_100MW_35MVAr : spsThreePhaseSeriesRLCLoadLib/Three-Phase Series RLC Load  LConnTagsString=A|B|C  Configuration=Y (grounded)  NominalVoltage=(230000)*0.948799  Vabc=[1e3 1e3 1e3]  Vabcp=[1e3 1e3 1e3]  NominalFrequency=60  UnbalancedPower=off  ActivePower=100000000  InductivePower=35000000  CapacitivePower=0  Pabc=[10e3 9e3 11e3]  QLabc=[100 90 110]  QCabc=[100 90 110]  Pabcp=[10e3 9e3 11e3]  QLabcp=[100 90 110]  QCabcp=[100 90 110]  Measurements=None  LoadType=constant PQ
  Line_4_5 : spsThreePhasePISectionLineLib/Three-Phase PI Section Line  LConnTagsString=a|b|c  RConnTagsString=A|B|C  Length=50  Frequency=60  Resistances=[ 0.199333 0.3864]  Inductances="[ 2.9658e-3  4.1264e-3]"  Capacitances=[7.751e-9 7.751e-9]
  Line_4_6 : spsThreePhasePISectionLineLib/Three-Phase PI Section Line  LConnTagsString=a|b|c  RConnTagsString=A|B|C  Length=50  Frequency=60  Resistances=[ 0.248707 0.3864]  Inductances="[ 3.0967e-3  4.1264e-3]"  Capacitances=[7.751e-9 7.751e-9]
  Line_5_7 : spsThreePhasePISectionLineLib/Three-Phase PI Section Line  LConnTagsString=a|b|c  RConnTagsString=A|B|C  Length=100  Frequency=60  Resistances=[ 0.24165 0.3864]  Inductances="[ 2.8816e-3  4.1264e-3]"  Capacitances=[7.751e-9 7.751e-9]
  Line_6_9 : spsThreePhasePISectionLineLib/Three-Phase PI Section Line  LConnTagsString=a|b|c  RConnTagsString=A|B|C  Length=100  Frequency=60  Resistances=[ 0.26634 0.3864]  Inductances="[ 2.9658e-3  4.1264e-3]"  Capacitances=[7.751e-9 7.751e-9]
  Line_7_8 : spsThreePhasePISectionLineLib/Three-Phase PI Section Line  LConnTagsString=a|b|c  RConnTagsString=A|B|C  Length=50  Frequency=60  Resistances=[ 0.18875 0.3864]  Inductances="[ 2.7226e-3  4.1264e-3]"  Capacitances=[6.751e-9 7.751e-9]
  Line_8_9 : spsThreePhasePISectionLineLib/Three-Phase PI Section Line  LConnTagsString=a|b|c  RConnTagsString=A|B|C  Length=100  Frequency=60  Resistances=[ 0.17077 0.3864]  Inductances="[ 2.3184e-3  4.1264e-3]"  Capacitances=[7.751e-9 7.751e-9]
  Load Flow Bus : spsLoadFlowBusLib/Load Flow Bus  LConnTagsString=a  Phases=single  Connectors=on one side  ID=BUS_3  Vbase=13.8e3  Vref=1  Vangle=0  VLF=1  VLFb=1  VLFc=1  angleLF=-0.3643  angleLFb=0  angleLFc=0
  Load Flow Bus1 : spsLoadFlowBusLib/Load Flow Bus  LConnTagsString=a  Phases=single  Connectors=on one side  ID=BUS_2  Vbase=18e3  Vref=1  Vangle=0  VLF=1  VLFb=1  VLFc=1  angleLF=6.369  angleLFb=0  angleLFc=0
  Load Flow Bus2 : spsLoadFlowBusLib/Load Flow Bus  LConnTagsString=a  Phases=single  Connectors=on one side  ID=BUS_1  Vbase=16.5e3  Vref=1  Vangle=0  VLF=1  VLFb=1  VLFc=1  angleLF=0  angleLFb=0  angleLFc=0
  Load Flow Bus3 : spsLoadFlowBusLib/Load Flow Bus  LConnTagsString=a  Phases=single  Connectors=on one side  ID=BUS_4  Vbase=230e3  Vref=1  Vangle=0  VLF=0.9522  VLFb=1  VLFc=1  angleLF=23.85  angleLFb=0  angleLFc=0
  Load Flow Bus4 : spsLoadFlowBusLib/Load Flow Bus  LConnTagsString=a  Phases=single  Connectors=on one side  ID=BUS_5  Vbase=230e3  Vref=1  Vangle=0  VLF=0.9038  VLFb=1  VLFc=1  angleLF=20.7  angleLFb=0  angleLFc=0
  Load Flow Bus5 : spsLoadFlowBusLib/Load Flow Bus  LConnTagsString=a  Phases=single  Connectors=on one side  ID=BUS_7  Vbase=230e3  Vref=1  Vangle=0  VLF=0.9761  VLFb=1  VLFc=1  angleLF=30.39  angleLFb=0  angleLFc=0
  Load Flow Bus6 : spsLoadFlowBusLib/Load Flow Bus  LConnTagsString=a  Phases=single  Connectors=on one side  ID=BUS_8  Vbase=230e3  Vref=1  Vangle=0  VLF=0.9488  VLFb=1  VLFc=1  angleLF=25.46  angleLFb=0  angleLFc=0
  Load Flow Bus7 : spsLoadFlowBusLib/Load Flow Bus  LConnTagsString=a  Phases=single  Connectors=on one side  ID=BUS_9  Vbase=230e3  Vref=1  Vangle=0  VLF=0.9844  VLFb=1  VLFc=1  angleLF=26.79  angleLFb=0  angleLFc=0
  Load Flow Bus8 : spsLoadFlowBusLib/Load Flow Bus  LConnTagsString=a  Phases=single  Connectors=on one side  ID=BUS_6  Vbase=230e3  Vref=1  Vangle=0  VLF=0.9163  VLFb=1  VLFc=1  angleLF=18.51  angleLFb=0  angleLFc=0
  M1 : spsSynchronousMachinepuStandardLib/Synchronous Machine pu Standard  PresetModel=No  MechanicalLoad=Mechanical power Pm  ShowDetailedParameters=on  RotorType=Salient-pole  Units=per unit standard parameters  MeasurementBus=off  NominalParameters="[200E6  16500   60 ]"  Reactances1=[ 31 32 33 34 35 36 37 ]  Reactances2=[ 1.305, 0.296, 0.252, 0.474, 0.243, 0.18 ]  dAxisTimeConstants=Short-circuit  qAxisTimeConstants=Short-circuit  TimeConstants1=[]  TimeConstants2=[]  TimeConstants3=[]  TimeConstants4=[]  TimeConstants5=[ 1.01, 0.053, 0.1 ]  TimeConstants6=[]  TimeConstants7=[ 1.01, 0.053, 0.0513 ]  TimeConstants8=[]  StatorResistance=2.8544e-3  Mechanical="[ 3.7 0  32]"  PolePairs=32  InitialConditions=[0 -74.864 0.725613 0.725613 0.725613 -25.1286 -145.129 94.8714 1.5789]  SetSaturation=off  Saturation=[0.6404,0.7127,0.8441,0.9214,0.9956,1.082,1.19,1.316,1.457;0.7,0.7698,0.8872,0.9466,0.9969,1.046,1.1,1.151,1.201]  LoadFlowParameters=[2 4000000000 0 0]  TsPowergui=0  TsBlock=-1  IterativeModel=Trapezoidal non iterative  IterativeDiscreteModel=Trapezoidal robust  BusType=swing  Pref=0  Qref=0  Qmin=-Inf  Qmax=Inf  PLF=0  QLF=0
  M2 : spsSynchronousMachinepuStandardLib/Synchronous Machine pu Standard  PresetModel=No  MechanicalLoad=Mechanical power Pm  ShowDetailedParameters=on  RotorType=Salient-pole  Units=per unit standard parameters  MeasurementBus=off  NominalParameters="[200E6  18000   60 ]"  Reactances1=[ 31 32 33 34 35 36 37 ]  Reactances2=[ 1.305, 0.296, 0.252, 0.474, 0.243, 0.18 ]  dAxisTimeConstants=Short-circuit  qAxisTimeConstants=Short-circuit  TimeConstants1=[]  TimeConstants2=[]  TimeConstants3=[]  TimeConstants4=[]  TimeConstants5=[ 1.01, 0.053, 0.0513 ]  TimeConstants6=[]  TimeConstants7=[ 1.01, 0.053, 0.0513 ]  TimeConstants8=[]  StatorResistance=2.8544e-3  Mechanical="[ 3.7 0  32]"  PolePairs=32  InitialConditions=[0 -64.2127 0.85432 0.85432 0.85432 -8.68499 -128.685 111.315 1.57616]  SetSaturation=off  Saturation=[0.6404,0.7127,0.8441,0.9214,0.9956,1.082,1.19,1.316,1.457;0.7,0.7698,0.8872,0.9466,0.9969,1.046,1.1,1.151,1.201]  LoadFlowParameters=[1 950000000 0 0]  TsPowergui=0  TsBlock=-1  IterativeModel=Trapezoidal non iterative  IterativeDiscreteModel=Trapezoidal robust  BusType=PV  Pref=165000000  Qref=0  Qmin=-Inf  Qmax=Inf  PLF=0  QLF=0
  M3 : spsSynchronousMachinepuStandardLib/Synchronous Machine pu Standard  PresetModel=No  MechanicalLoad=Mechanical power Pm  ShowDetailedParameters=on  RotorType=Salient-pole  Units=per unit standard parameters  MeasurementBus=off  NominalParameters="[200E6  13.8e3   60 ]"  Reactances1=[ 31 32 33 34 35 36 37 ]  Reactances2=[ 1.305, 0.296, 0.252, 0.474, 0.243, 0.18 ]  dAxisTimeConstants=Short-circuit  qAxisTimeConstants=Short-circuit  TimeConstants1=[]  TimeConstants2=[]  TimeConstants3=[]  TimeConstants4=[]  TimeConstants5=[ 1.01, 0.053, 0.1 ]  TimeConstants6=[]  TimeConstants7=[ 1.01, 0.053, 0.0513 ]  TimeConstants8=[]  StatorResistance=2.8544e-3  Mechanical="[ 3.7 0  32]"  PolePairs=32  InitialConditions=[0 -79.6776 0.446083 0.446083 0.446083 -18.0501 -138.05 101.95 1.26041]  SetSaturation=off  Saturation=[0.6404,0.7127,0.8441,0.9214,0.9956,1.082,1.19,1.316,1.457;0.7,0.7698,0.8872,0.9466,0.9969,1.046,1.1,1.151,1.201]  LoadFlowParameters=[1 950000000 0 0]  TsPowergui=0  TsBlock=-1  IterativeModel=Trapezoidal non iterative  IterativeDiscreteModel=Trapezoidal robust  BusType=PV  Pref=85000000  Qref=0  Qmin=-Inf  Qmax=Inf  PLF=0  QLF=0
  MATLAB Function1 : MATLAB Function  TreatAsAtomicUnit=on  mask{N=N}
      mask prompts: N "Harmonic order:"
  MATLAB Function2 : MATLAB Function  TreatAsAtomicUnit=on  mask{N=N}
      mask prompts: N "Harmonic order:"
  MATLAB Function3 : MATLAB Function  TreatAsAtomicUnit=on  mask{N=N}
      mask prompts: N "Harmonic order:"
  MATLAB Function4 : MATLAB Function  TreatAsAtomicUnit=on  mask{N=N}
      mask prompts: N "Harmonic order:"
  MATLAB Function5 : MATLAB Function  TreatAsAtomicUnit=on  mask{N=N}
      mask prompts: N "Harmonic order:"
  MATLAB Function6 : MATLAB Function  TreatAsAtomicUnit=on  mask{N=N}
      mask prompts: N "Harmonic order:"
  MatMux1 : Subsystem  mask{nrInp=3}
      mask prompts: nrInp "Number of inputs [{C}]"
      mask init:
      | %blocks = find_system(gcb,'LookUnderMasks','on','FollowLinks','on')
      | %set_param(gcb, 'MaskSelfModifiable', 'on');
      | 
      | % if(SSM == [])
      | %     Simulink.SubSystem.deleteContents(gcb);
      | % else
      | 
      | if(isempty(nrInp))
      |     Simulink.SubSystem.deleteContents(gcb);
      | else
      | 
      |     nrOut = 1;
      | 
      | 
      | PortHandles = get_param(gcb,'PortHandles');
      | lenInp = length(PortHandles.Inport);
      | lenOut = length(PortHandles.Inport);
      | 
      | if(nrInp ~= lenInp)
      |     %disp('ENTERED')
      |     Simulink.SubSystem.deleteContents(gcb);
      | %     add_block('simulink/Continuous/State-Space', [gcb,'/ss_block'], 'A','SS.A', 'B','SS.B', 'C','SS.C', 'D','SS.D', 'X0','X0')
      | %     set_param([gcb,'/ss_block'],'position' , [350,100,450,150])
      | 
      | 
      | 
      |         add_block('simulink/Math Operations/Matrix Concatenate',[gcb,'/Mux'], 'NumInputs',num2str(nrInp), 'ConcatenateDimension',num2str(2));
      |         set_param([gcb,'/Mux'],'position' , [200,100,250,100+nrInp*50])
      |         
      | %         add_block('built-in/Demux',[gcb,'/Demux'], 'Outputs',num2str(nrOut));
      | %         set_param([gcb,'/Demux'],'position' , [500,100,550,100+nrOut*50])
      | 
      | 
      |         for i = 1 : nrInp
      |             add_block('built-in/Inport',[gcb,strcat('/In',num2str(i))]);
      |             set_param([gcb,strcat('/In',num2str(i))],'position' , [50,65+i*50,90,85+i*50]);
      |             add_line(gcb,strcat('In',num2str(i),'/1'),strcat('Mux/',num2str(i)),'autorouting','on');
      |         end
      | 
      |         for i = 1 : nrOut
      |             add_block('built-in/Outport',[gcb,strcat('/Out',num2str(i))]);
      |             set_param([gcb,strcat('/Out',num2str(i))],'position' , [750,65+i*50,790,85+i*50]);
      |             add_line(gcb,strcat('Mux/',num2str(i)), strcat('Out',num2str(i),'/1'),'autorouting','on');
      |         end
      | 
      | 
      | %     add_line(gcb, 'Mux/1', 'ss_block/1')
      | %     add_line(gcb, 'ss_block/1', 'Demux/1')
      | 
      | end
      | 
      | end
      mask Display: disp(['{\color{red}\bf\fontsize{12}} [\{C\}]',newline,' MUX'], 'texmode','on');
  MatMux2 : Subsystem  mask{nrInp=3}
      mask prompts: nrInp "Number of inputs [{C}]"
      mask init: same as IEEE_9bus/MatMux1
      mask Display: disp(['{\color{red}\bf\fontsize{12}} [\{C\}]',newline,' MUX'], 'texmode','on');
  MatMux3 : Subsystem  Commented=on  mask{nrInp=3}
      mask prompts: nrInp "Number of inputs [{C}]"
      mask init: same as IEEE_9bus/MatMux1
      mask Display: disp(['{\color{red}\bf\fontsize{12}} [\{C\}]',newline,' MUX'], 'texmode','on');
  Mux : Mux  Commented=on  Inputs=3
  Mux1 : Mux  Commented=on  Inputs=3
  Mux{5..18} (14 alike) : Mux  Inputs=2
  Mux2 : Mux  Commented=on  Inputs=2
  Mux3 : Mux  Commented=on  Inputs=2
  Mux4 : Mux  Commented=on  Inputs=2
  Mux53 : Mux  Inputs=3
  Mux54 : Mux  Inputs=3
  Mux55 : Mux  Inputs=3
  "PMU (PLL-Based, Positive-Sequence)" : spsPMUPLLBasedPositiveSequenceLib/PMU (PLL-Based, Positive-Sequence)  Commented=on  nominalFrequency=60  samplingRate=64  reportingFactor=1
      settings: LibrarySourceBlock=|
      | sps_lib/Sensors and Measurements/PMU
      | (PLL-Based,
      | Positive-Sequence)
  PSS selector{,2..4} (4 alike) : ManualSwitch  CurrentSetting=0
  PSS selector{1,5..8} (5 alike) : ManualSwitch
  PSS selector9 : ManualSwitch  Commented=on  CurrentSetting=0
  SS_DelayPrediction : Subsystem  Commented=on  mask{N=N, Ts=Ts, x0=SYS.x0}
      mask prompts: N "Order number:"; Ts "Time step (s):"; x0 "Initial conditions (x0):"
      mask init:
      | a = -0.5+0.866i;
      | a2 = -0.5-0.866i;
      | Sas = [1,a,a2;1,a2,a;1,1,1]/3;
      | 
      | Zpnz_old = complex(zeros(size(x0,1),N+1));
      | 
      | if(~isempty(x0))
      | 
      |     if(mod(numel(x0),3)~=0) error('[Delay predictor] x0 vector with wrong size --> needs to be a multiple of 3!'); end
      | 
      |     for k = 1 : numel(x0)/3
      |         Zpnz_old((k-1)*3+1:(k-1)*3+3,1) = Sas*x0((k-1)*3+1:(k-1)*3+3);
      |     end
      | end
  Scope : Scope  Commented=on  NumInputPorts=3
  Scope1 : Scope
  Scope3 : Scope
  Selector{1..6} (6 alike) : Selector  InputPortWidth=3  IndexOptions=Index vector (dialog)  Indices=[1 2]  OutputSizes=1
  Subsystem : Subsystem
  TR_1_4 : spsThreePhaseTransformerTwoWindingsLib/Three-Phase Transformer (Two Windings)  Winding1Connection=Delta (D1)  Winding2Connection=Yg  CoreType=Three single-phase transformers  SetSaturation=off  Hysteresis=off  DataFile='hysteresis'  SetInitialFlux=off  Measurements=None  UNITS=pu  NominalPower=[ 200e6 , 60 ]  Winding1=[ 16.5e3 , 0.002 , 0.08 ]  Winding2=[ 230e3 , 0.002 , 0.08 ]  Rm=500  Lm=500  L0=0.5  Saturation=[ 0,0 ; 0.0024,1.2 ; 1.0,1.52 ]  InitialFluxes=[ 0.8 , -0.8 , 0.7 ]  BreakLoop=off  DiscreteSolver=Trapezoidal iterative  DataType=off  TransfoNumber=1
  TR_2_7 : spsThreePhaseTransformerTwoWindingsLib/Three-Phase Transformer (Two Windings)  Winding1Connection=Delta (D1)  Winding2Connection=Yg  CoreType=Three single-phase transformers  SetSaturation=off  Hysteresis=off  DataFile='hysteresis'  SetInitialFlux=off  Measurements=None  UNITS=pu  NominalPower=[ 100e6 , 60 ]  Winding1=[ 18e3 , 1e-4 , 0.0625/2 ]  Winding2=[ 230e3 , 1e-4 , 0.0625/2 ]  Rm=500  Lm=500  L0=0.5  Saturation=[ 0,0 ; 0.0024,1.2 ; 1.0,1.52 ]  InitialFluxes=[ 0.8 , -0.8 , 0.7 ]  BreakLoop=off  DiscreteSolver=Trapezoidal iterative  DataType=off  TransfoNumber=1
  TR_3_9 : spsThreePhaseTransformerTwoWindingsLib/Three-Phase Transformer (Two Windings)  Winding1Connection=Delta (D1)  Winding2Connection=Yg  CoreType=Three single-phase transformers  SetSaturation=off  Hysteresis=off  DataFile='hysteresis'  SetInitialFlux=off  Measurements=None  UNITS=pu  NominalPower=[ 100e6 , 60 ]  Winding1=[ 13.8e3 , 1e-4 , 0.0586/2 ]  Winding2=[ 230e3 , 1e-4 , 0.0586/2 ]  Rm=500  Lm=500  L0=0.5  Saturation=[ 0,0 ; 0.0024,1.2 ; 1.0,1.52 ]  InitialFluxes=[ 0.8 , -0.8 , 0.7 ]  BreakLoop=off  DiscreteSolver=Trapezoidal iterative  DataType=off  TransfoNumber=1
  Three-Phase V-I Measurement1 : spsThreePhaseVIMeasurementLib/Three-Phase V-I Measurement  VoltageMeasurement=phase-to-phase  SetLabelV=on  LabelV=Vabc_B6  Vpu=off  VpuLL=on  CurrentMeasurement=no  SetLabelI=off  LabelI=Iabc  Ipu=off  Pbase=100e6  Vbase=230e3  OutputType=Complex  PhasorSimulation=off  PSBequivalent=0
  Three-Phase V-I Measurement2 : spsThreePhaseVIMeasurementLib/Three-Phase V-I Measurement  VoltageMeasurement=phase-to-phase  SetLabelV=on  LabelV=Vabc_B9  Vpu=off  VpuLL=on  CurrentMeasurement=no  SetLabelI=off  LabelI=Iabc  Ipu=off  Pbase=100e6  Vbase=230e3  OutputType=Complex  PhasorSimulation=off  PSBequivalent=0
  Three-Phase Fault : spsThreePhaseFaultLib/Three-Phase Fault  Commented=on  InitialStates=0  FaultA=on  FaultB=on  FaultC=on  GroundFault=on  SwitchTimes=[24 24.1]  External=off  SwitchStatus=NaN  FaultResistance=0.001  GroundResistance=0.01  SnubberResistance=1e6  SnubberCapacitance=inf  Measurements=None
  Turbine & Regulators M1 : Subsystem
  Turbine & Regulators M1c : Subsystem
  Turbine & Regulators M2 : Subsystem
  Turbine & Regulators M2c : Subsystem
  Turbine & Regulators M3 : Subsystem
  Turbine & Regulators M3c : Subsystem
  V-I Meas Bus 1 : spsThreePhaseVIMeasurementLib/Three-Phase V-I Measurement  VoltageMeasurement=phase-to-ground  SetLabelV=on  LabelV=VBUS1  Vpu=off  VpuLL=off  CurrentMeasurement=yes  SetLabelI=on  LabelI=IBUS1  Ipu=off  Pbase=100e6  Vbase=500e3  OutputType=Complex  PhasorSimulation=off  PSBequivalent=0
  V-I Meas Bus 2 : spsThreePhaseVIMeasurementLib/Three-Phase V-I Measurement  VoltageMeasurement=phase-to-ground  SetLabelV=on  LabelV=VBUS2  Vpu=off  VpuLL=off  CurrentMeasurement=yes  SetLabelI=on  LabelI=IBUS2  Ipu=off  Pbase=100e6  Vbase=500e3  OutputType=Complex  PhasorSimulation=off  PSBequivalent=0
  V-I Meas Bus 3 : spsThreePhaseVIMeasurementLib/Three-Phase V-I Measurement  VoltageMeasurement=phase-to-ground  SetLabelV=on  LabelV=VBUS3  Vpu=off  VpuLL=off  CurrentMeasurement=yes  SetLabelI=on  LabelI=IBUS3  Ipu=off  Pbase=100e6  Vbase=500e3  OutputType=Complex  PhasorSimulation=off  PSBequivalent=0
  XY{,3..4,6} (4 alike) : Scope  NumInputPorts=3
  XY1 : Scope  Commented=on  NumInputPorts=3
  XY2 : Scope  NumInputPorts=5
  abc to dq{1..5,7} (6 alike) : spsabctodq0Lib/abc to dq0  Alignment=90 degrees behind phase A axis
  powergui : sps_lib/powergui  Priority=1  SimulationMode=Discrete  SampleTime=Ts  frequency=60  Iterations=50  frequencyindice=60  Pbase=200  ErrMax=0.0001  UnitsV=kV  UnitsW=MW  buscounter=0  FunctionMessages=off  echomessages=off  EnableUseOfTLC=off  CurrentSourceSwitches=off  DisableSnubberDevices=off  DisableRonSwitches=off  DisableVfSwitches=off  DisplayEquations=off  AutomaticDiscreteSolvers=off  SolverType=Tustin/Backward Euler (TBE)  Interpol=off  ExternalGateDelay=off  methode=off  Ts=100  x0status=blocks  SPID=on  SwTol=0  HookPort=off  NonlinearTolerance=1e-4  nMaxIteration=100  ContinueOnMaxIteration=off  RestoreLinks=warning  ResistiveCurrentMeasurement=off  Frange=[0:2:500]  Ylog=off  Xlog=on  ShowGrid=off  save=off  variable=ZData  structure=0  ZoomFFT=off  StartTime=0.0  cycles=1  DisplayStyle=1  fundamental=60  FreqAxis=off  MaxFrequency=1000  frequencyindicesteady=1  RmsSteady=1  display=off
  tag scope: PSS=global
  wires:
  From/1 -> "PMU (PLL-Based, Positive-Sequence)"/1
  "PMU (PLL-Based, Positive-Sequence)"/3 -> Scope/3
  "PMU (PLL-Based, Positive-Sequence)"/2 -> Scope/2
  "PMU (PLL-Based, Positive-Sequence)"/1 -> Scope/1
  Turbine & Regulators M1/2(Vf) -> [Vf1], M1/2
  Turbine & Regulators M1/1(Pm) -> [Pm1], M1/1
  Constant/1 -> [Pref1], Turbine & Regulators M1/2(Pref)
  PSS selector/1 -> PSS selector1/1
  Subsystem/1(Generic) -> PSS selector/1
  Subsystem/3(No PSS) -> PSS selector1/2
  Subsystem/2(Multiband) -> PSS selector/2
  PSS selector1/1 -> [PSS]
  Constant1/1 -> [Pref2], Turbine & Regulators M2/2(Pref)
  Turbine & Regulators M2/1(Pm) -> [Pm2], M2/1
  Turbine & Regulators M2/2(Vf) -> [Vf2], M2/2
  Turbine & Regulators M3/2(Vf) -> [Vf3], M3/2
  Turbine & Regulators M3/1(Pm) -> [Pm3], M3/1
  Constant2/1 -> [Pref3], Turbine & Regulators M3/2(Pref)
  [Vabc_B9] -> Scope1/1
  M1/1 -> [m1]
  [m1] -> Turbine & Regulators M1/1(m)
  M3/1 -> [m3]
  [m3] -> Turbine & Regulators M3/1(m)
  M2/1 -> [m2]
  [m2] -> Turbine & Regulators M2/1(m)
  Discrete State-Space1/1 -> Gain1/1
  From5/1 -> ABsel/1(In1)
  From6/1 -> ABsel1/1(In1)
  From7/1 -> ABsel2/1(In1)
  Demux/1 -> Goto4/1
  Demux/2 -> Goto5/1
  Demux/3 -> Goto6/1
  DQn->ABC4/1(Xabc) -> Gain/1
  Gain/1 -> Demux11/1
  ABsel/1(Out1) -> Mux/1
  ABsel1/1(Out1) -> Mux/2
  ABsel2/1(Out1) -> Mux/3
  DQN_Mac2_V1/1 -> [Im2_C]
  PSS selector3/1 -> DQN_Mac2_V1/1
  abc to dq7/1 -> Selector6/1  "vq,vd"
  [theta0] -> abc to dq7/2  "theta"
  Selector6/1 -> MATLAB Function5/1(Vdq_vec)
  MATLAB Function5/1(Vs_c) -> PSS selector3/1  "[N+1,18 (6+6+6)]"
  ? -> [theta_m2]
  Selector1/1 -> MATLAB Function1/1(Vdq_vec)
  abc to dq1/1 -> Selector1/1  "vq,vd"
  MATLAB Function1/1(Vs_c) -> PSS selector2/1  "[N+1,18 (6+6+6)]"
  [theta0] -> abc to dq1/2  "theta"
  Selector2/1 -> MATLAB Function2/1(Vdq_vec)
  abc to dq2/1 -> Selector2/1  "vq,vd"
  MATLAB Function2/1(Vs_c) -> PSS selector4/1  "[N+1,18 (6+6+6)]"
  [IBUS2] -> Gain5/1
  Demux6/2 -> Mux7/1  "Mac_EMT_b"
  Mux7/1 -> XY3/2
  Demux5/3 -> Mux8/2  "Mac_SS_c"
  Demux6/1 -> Mux9/1  "Mac_EMT_a"
  Mux9/1 -> XY3/1
  Demux5/1 -> Mux9/2  "Mac_SS_a"
  Mux8/1 -> XY3/3
  Demux6/3 -> Mux8/1  "Mac_EMT_c"
  Demux5/2 -> Mux7/2  "Mac_SS_b"
  DQn->ABC1/1(Xabc) -> [Im2_abc], Demux5/1
  Mux10/1 -> XY4/2
  DQn->ABC3/1(Xabc) -> [Im1_abc], Demux7/1
  Demux7/2 -> Mux10/2  "Mac_SS_b"
  Mux11/1 -> XY4/3
  Mux12/1 -> XY4/1
  Demux8/3 -> Mux11/1  "Mac_EMT_c"
  Demux7/1 -> Mux12/2  "Mac_SS_a"
  Demux7/3 -> Mux11/2  "Mac_SS_c"
  Demux8/2 -> Mux10/1  "Mac_EMT_b"
  [IBUS1] -> Gain4/1
  Demux8/1 -> Mux12/1  "Mac_EMT_a"
  DQN_Mac1_V1/1(I_C) -> [Im1_C]
  PSS selector2/1 -> DQN_Mac1_V1/1(Vs_C)
  Mux13/1 -> XY6/2
  DQn->ABC2/1(Xabc) -> [Im3_abc], Demux9/1
  Demux9/2 -> Mux13/2  "Mac_SS_b"
  Mux14/1 -> XY6/3
  Mux15/1 -> XY6/1
  Demux10/3 -> Mux14/1  "Mac_EMT_c"
  Demux9/1 -> Mux15/2  "Mac_SS_a"
  Demux9/3 -> Mux14/2  "Mac_SS_c"
  Demux10/2 -> Mux13/1  "Mac_EMT_b"
  [IBUS3] -> Gain6/1
  Demux10/1 -> Mux15/1  "Mac_EMT_a"
  PSS selector4/1 -> DQN_Mac3_V1/1
  Clock/1 -> Gain12/1
  Gain12/1 -> [theta0]
  [theta0] -> DQn->ABC4/2(tho)
  [VBUS1_C] -> DQn->ABC4/1(Xdcpnz_c)
  [VBUS1_C] -> PSS selector2/2
  [VBUS2_C] -> PSS selector3/2
  [VBUS3_C] -> PSS selector4/2
  DQN_Mac3_V1/1 -> [Im3_C]
  DQN_Mac3_V1/2 -> Turbine & Regulators M3c/2(m)
  [theta0] -> DQn->ABC3/2(tho)
  [Im1_C] -> DQn->ABC3/1(Xdcpnz_c)
  [Im2_C] -> DQn->ABC1/1(Xdcpnz_c)
  [theta0] -> DQn->ABC1/2(tho)
  [Im3_C] -> DQn->ABC2/1(Xdcpnz_c)
  [theta0] -> DQn->ABC2/2(tho)
  Mux54/1 -> XY/2
  Mux55/1 -> XY/3
  Demux46/1 -> Mux53/2  "Mac_SS_a"
  Demux47/2 -> Mux54/1  "Mac_EMT_b"
  Demux11/2 -> Mux54/3  "Mac_DQN_b"
  Mux53/1 -> XY/1
  Demux11/3 -> Mux55/3  "Mac_DQN_c"
  Demux47/1 -> Mux53/1  "Mac_EMT_a"
  Demux46/2 -> Mux54/2  "Mac_SS_b"
  Demux46/3 -> Mux55/2  "Mac_SS_c"
  Demux11/1 -> Mux53/3  "Mac_DQN_a"
  Demux47/3 -> Mux55/1  "Mac_EMT_c"
  [VBUS1] -> Demux47/1
  [VBUS1_SS] -> Demux46/1
  [theta0] -> abc to dq2/2  "theta"
  PSS selector5/1 -> abc to dq1/1
  [VBUS1] -> PSS selector5/1  "v"
  PSS selector6/1 -> abc to dq7/1
  [VBUS2] -> PSS selector6/1  "v"
  PSS selector7/1 -> abc to dq2/1
  [VBUS3] -> PSS selector7/1  "v"
  [VBUS1_SS] -> PSS selector5/2
  [VBUS2_SS] -> PSS selector6/2
  [VBUS3_SS] -> PSS selector7/2
  Gain1/1 -> Demux/1
  [Im1_C] -> MatMux2/1(In1)
  [Im2_C] -> MatMux2/2(In2)
  [Im3_C] -> MatMux2/3(In3)
  Demux_DQNc_Mat/1(Out1) -> [VBUS1_C]
  Demux_DQNc_Mat/2(Out2) -> [VBUS2_C]
  Demux_DQNc_Mat/3(Out3) -> [VBUS3_C]
  abc to dq3/1 -> Selector3/1  "vq,vd"
  [IBUS1] -> abc to dq3/1
  [theta0] -> abc to dq3/2  "theta"
  Selector3/1 -> MATLAB Function3/1(Vdq_vec)
  abc to dq4/1 -> Selector4/1  "vq,vd"
  Selector4/1 -> MATLAB Function4/1(Vdq_vec)
  [IBUS2] -> abc to dq4/1
  [theta0] -> abc to dq4/2  "theta"
  MATLAB Function4/1(Vs_c) -> MatMux1/2(In2)  "[N+1,18 (6+6+6)]"
  Selector5/1 -> MATLAB Function6/1(Vdq_vec)
  [IBUS3] -> abc to dq5/1
  [theta0] -> abc to dq5/2  "theta"
  abc to dq5/1 -> Selector5/1  "vq,vd"
  MATLAB Function6/1(Vs_c) -> MatMux1/3(In3)  "[N+1,18 (6+6+6)]"
  MATLAB Function3/1(Vs_c) -> MatMux1/1(In1)  "[N+1,18 (6+6+6)]"
  Gain_DQNc_Mat1/1 -> Demux_DQNc_Mat2/1(In1)
  Gain_DQNc_Mat4/1(Ypnz) -> Add3/1
  Int_DQNc_Mat3/1(Zpnz) -> SS_DelayPrediction/1(in)  "dw"
  Demux_DQNc_Mat2/2(Out2) -> Goto13/1
  Gain_DQNc_Mat5/1 -> Add3/2  "dw"
  SS_DelayPrediction/1(dw) -> Gain_DQNc_Mat5/1, Gain_DQNc_Mat1/1  "dw"
  Demux_DQNc_Mat2/3(Out3) -> Goto14/1
  Add3/1 -> Int_DQNc_Mat3/1(Xpnz)  "dw"
  Demux_DQNc_Mat2/1(Out1) -> Goto10/1
  MatMux2/1(Out1) -> Gain8/1
  PSS selector8/1 -> Gain7/1
  Discrete State-Space2/1(Y) -> Scope3/1, Demux_DQNc_Mat/1(In1)
  PSS selector9/1 -> Discrete State-Space1/1
  Mux/1 -> PSS selector9/2
  From50/1 -> Mux1/2
  From53/1 -> Mux1/3
  From48/1 -> Mux1/1
  Mux1/1 -> PSS selector9/1
  [VBUS1] -> ABsel3/1(In1)  "v"
  Demux1/3 -> Mux3/2  "Mac_SS_c"
  Mux2/1 -> XY1/2
  Demux1/1 -> Mux4/2  "Mac_SS_a"
  Demux2/1 -> Mux4/1  "Mac_EMT_a"
  Demux1/2 -> Mux2/2  "Mac_SS_b"
  Demux2/3 -> Mux3/1  "Mac_EMT_c"
  Mux3/1 -> XY1/3
  Mux4/1 -> XY1/1
  From56/1 -> Demux2/1
  Demux2/2 -> Mux2/1  "Mac_EMT_b"
  Gain3/1 -> Demux1/1
  ABsel4/1(Out1) -> Gain3/1
  ABsel3/1(Out1) -> ?
  Gain2/1 -> Discrete State-Space3/1(U)
  Turbine & Regulators M2c/1(Vf) -> DQN_Mac2_V1/2
  Turbine & Regulators M2c/2(Pm) -> DQN_Mac2_V1/3
  Turbine & Regulators M3c/1(Pm) -> DQN_Mac3_V1/2
  Turbine & Regulators M3c/2(Vf) -> DQN_Mac3_V1/3
  Gain4/1 -> Demux8/1
  Gain5/1 -> Demux6/1
  Gain6/1 -> Demux10/1
  Gain7/1 -> Discrete State-Space2/1(U)
  From58/1 -> MatMux3/3(In3)
  From55/1 -> MatMux3/1(In1)
  From57/1 -> MatMux3/2(In2)
  MatMux3/1(Out1) -> Gain9/1
  MatMux1/1(Out1) -> PSS selector8/2
  Gain8/1 -> PSS selector8/1
  Gain9/1 -> Gain_DQNc_Mat4/1(Xpnz)
  DQN_Mac1_V1/2(m) -> [m1c], Turbine & Regulators M1c/2(m)
  [m1] -> Bus Selector/1
  [m1c] -> Bus Selector1/1
  Mux6/1 -> XY2/3
  Mux16/1 -> XY2/1
  Mux5/1 -> XY2/2
  Mux18/1 -> XY2/5
  Bus Selector/1 -> Mux16/1  "<Stator voltage  vd (pu)>"
  Bus Selector1/1 -> Mux16/2  "<Stator voltage  vd (pu)>"
  Bus Selector/2 -> Mux5/1  "<Stator voltage  vq (pu)>"
  Bus Selector1/2 -> Mux5/2  "<Stator voltage  vq (pu)>"
  Bus Selector/3 -> Mux6/1  "<Rotor speed  wm  (pu)>"
  Bus Selector1/3 -> Mux6/2  "<Rotor speed  wm  (pu)>"
  Bus Selector1/4 -> Mux17/2  "<Rotor speed deviation  dw (pu)>"
  Bus Selector/4 -> Mux17/1  "<Rotor speed deviation  dw (pu)>"
  Mux17/1 -> XY2/4
  Bus Selector/5 -> Mux18/1  "<Output active power   Peo (pu)>"
  Bus Selector1/5 -> Mux18/2  "<Output active power   Peo (pu)>"
  Turbine & Regulators M1c/1(Vf) -> DQN_Mac1_V1/2(Vf)
  Turbine & Regulators M1c/2(Pm) -> DQN_Mac1_V1/3(Pm)
  [Pref1] -> Turbine & Regulators M1c/1(Pref)
  DQN_Mac2_V1/2 -> Turbine & Regulators M2c/2(m)
  [Pref2] -> Turbine & Regulators M2c/1(Pref)
  [Pref3] -> Turbine & Regulators M3c/1(Pref)
  connections:
  TR_1_4/RConn1 -- Load Flow Bus3/LConn1 -- Line_4_6/RConn1 -- Line_4_5/RConn1
  TR_1_4/RConn2 -- Line_4_6/RConn2 -- Line_4_5/RConn2
  TR_1_4/RConn3 -- Line_4_6/RConn3 -- Line_4_5/RConn3
  LD_6_50MW/LConn1 -- Line_6_9/RConn1 -- Load Flow Bus8/LConn1 -- Three-Phase V-I Measurement2/RConn1
  Line_4_6/LConn3 -- Three-Phase V-I Measurement2/LConn3 -- LD_6_90MW_30MVAr/LConn3
  Line_6_9/LConn1 -- Load Flow Bus7/LConn1 -- TR_3_9/RConn1 -- Line_8_9/RConn1
  Line_6_9/LConn2 -- TR_3_9/RConn2 -- Line_8_9/RConn2
  Line_6_9/LConn3 -- TR_3_9/RConn3 -- Line_8_9/RConn3
  Line_7_8/RConn1 -- LD_8_100MW_35MVAr/LConn1 -- Line_8_9/LConn1 -- Load Flow Bus6/LConn1
  Line_7_8/RConn2 -- LD_8_100MW_35MVAr/LConn2 -- Line_8_9/LConn2
  Line_7_8/RConn3 -- LD_8_100MW_35MVAr/LConn3 -- Line_8_9/LConn3
  Line_4_5/LConn1 -- Three-Phase Fault/LConn1 -- LD_5_125MW_50MVAr/LConn1 -- Load Flow Bus4/LConn1 -- Line_5_7/RConn1
  Line_4_5/LConn2 -- Three-Phase Fault/LConn2 -- LD_5_125MW_50MVAr/LConn2 -- Line_5_7/RConn2
  Line_4_5/LConn3 -- Three-Phase Fault/LConn3 -- LD_5_125MW_50MVAr/LConn3 -- Line_5_7/RConn3
  Three-Phase V-I Measurement1/RConn3 -- Line_5_7/LConn3 -- Line_7_8/LConn3
  Three-Phase V-I Measurement1/RConn2 -- Line_7_8/LConn2 -- Line_5_7/LConn2
  Three-Phase V-I Measurement1/RConn1 -- Load Flow Bus5/LConn1 -- Line_5_7/LConn1 -- Line_7_8/LConn1
  TR_2_7/RConn3 -- Three-Phase V-I Measurement1/LConn3
  TR_2_7/RConn2 -- Three-Phase V-I Measurement1/LConn2
  TR_2_7/RConn1 -- Three-Phase V-I Measurement1/LConn1
  Load Flow Bus/LConn1 -- V-I Meas Bus 3/LConn1 -- LD_3/LConn1 -- TR_3_9/LConn1
  LD_3/LConn2 -- V-I Meas Bus 3/LConn2 -- TR_3_9/LConn2
  TR_3_9/LConn3 -- V-I Meas Bus 3/LConn3 -- LD_3/LConn3
  V-I Meas Bus 2/LConn3 -- TR_2_7/LConn3 -- LD_2/LConn3
  V-I Meas Bus 2/LConn2 -- TR_2_7/LConn2 -- LD_2/LConn2
  Load Flow Bus1/LConn1 -- TR_2_7/LConn1 -- LD_2/LConn1 -- V-I Meas Bus 2/LConn1
  Load Flow Bus2/LConn1 -- LD_1/LConn1 -- V-I Meas Bus 1/LConn1 -- TR_1_4/LConn1
  V-I Meas Bus 1/LConn2 -- LD_1/LConn2 -- TR_1_4/LConn2
  V-I Meas Bus 1/LConn3 -- LD_1/LConn3 -- TR_1_4/LConn3
  LD_6_50MW/LConn3 -- Three-Phase V-I Measurement2/RConn3 -- Line_6_9/RConn3
  Line_4_6/LConn2 -- Three-Phase V-I Measurement2/LConn2 -- LD_6_90MW_30MVAr/LConn2
  Line_4_6/LConn1 -- Three-Phase V-I Measurement2/LConn1 -- LD_6_90MW_30MVAr/LConn1
  LD_6_50MW/LConn2 -- Three-Phase V-I Measurement2/RConn2 -- Line_6_9/RConn2
  V-I Meas Bus 3/RConn1 -- M3/RConn1
  V-I Meas Bus 3/RConn2 -- M3/RConn2
  V-I Meas Bus 3/RConn3 -- M3/RConn3
  M2/RConn1 -- V-I Meas Bus 2/RConn1
  M2/RConn2 -- V-I Meas Bus 2/RConn2
  M2/RConn3 -- V-I Meas Bus 2/RConn3
  M1/RConn1 -- V-I Meas Bus 1/RConn1
  M1/RConn2 -- V-I Meas Bus 1/RConn2
  M1/RConn3 -- V-I Meas Bus 1/RConn3
  Ground/LConn1 -- LD_2/RConn1 -- LD_2/RConn3 -- LD_2/RConn2
  Ground1/LConn1 -- LD_1/RConn1 -- LD_1/RConn3 -- LD_1/RConn2
  Ground2/LConn1 -- LD_3/RConn1 -- LD_3/RConn3 -- LD_3/RConn2
